simulink model "HW6_Q3"  (R2023a)
settings: Solver=VariableStepAuto  StartTime=0.0  StopTime=10  RelTol=1e-3
settings Model: Creator=USER  LastModifiedBy=USER

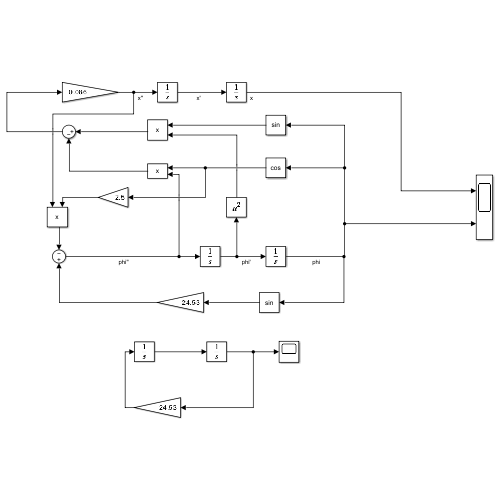
[thumbnail: Simulink's stored preview of the top-level diagram]
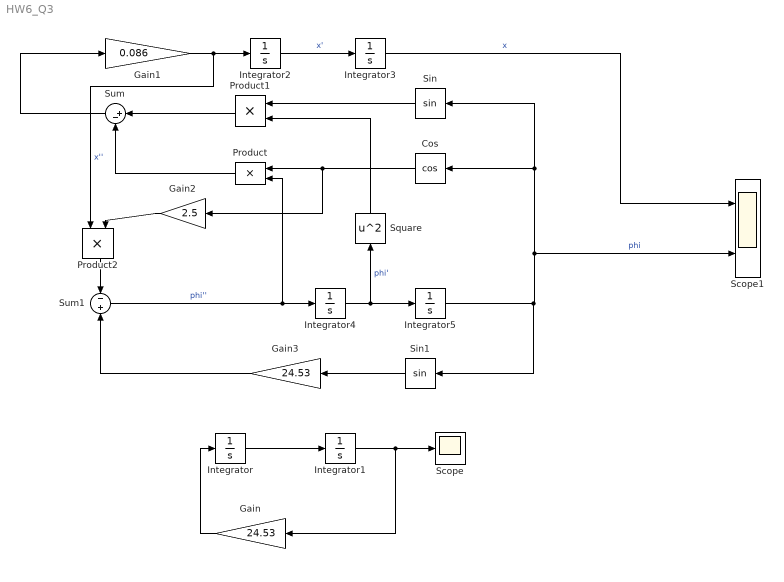
== system HW6_Q3 ==
  Cos : Trigonometry  Operator=cos
  Gain : Gain  Gain=24.53
  Gain1 : Gain  Gain=0.086
  Gain2 : Gain  Gain=2.5
  Gain3 : Gain  Gain=24.53
  Integrator : Integrator
  Integrator1 : Integrator  InitialCondition=0.1
  Integrator2 : Integrator
  Integrator3 : Integrator  InitialCondition=0.1
  Integrator4 : Integrator
  Integrator5 : Integrator  InitialCondition=0.1
  Product : Product
  Product1 : Product
  Product2 : Product
  Scope : Scope
  Scope1 : Scope  NumInputPorts=2
  Sin : Trigonometry
  Sin1 : Trigonometry
  Square : Math  Operator=square
  Sum : Sum  Inputs=|+-
  Sum1 : Sum  Inputs=-+
  wires:
  Integrator/1 -> Integrator1/1
  Integrator1/1 -> Gain/1, Scope/1
  Gain/1 -> Integrator/1
  Integrator2/1 -> Integrator3/1  "x'"
  Integrator4/1 -> Square/1, Integrator5/1  "phi'"
  Gain1/1 -> Product2/1, Integrator2/1  "x''"
  Integrator5/1 -> Sin1/1, Sin/1, Cos/1, Scope1/2  "phi"
  Sum1/1 -> Product/2, Integrator4/1  "phi''"
  Sum/1 -> Gain1/1
  Cos/1 -> Gain2/1, Product/1
  Product/1 -> Sum/2
  Sin/1 -> Product1/1
  Square/1 -> Product1/2
  Product1/1 -> Sum/1
  Integrator3/1 -> Scope1/1  "x"
  Product2/1 -> Sum1/1
  Gain2/1 -> Product2/2
  Sin1/1 -> Gain3/1
  Gain3/1 -> Sum1/2
